simulink model "test_ecef"  (R2019b)
settings: Solver=VariableStepAuto  StartTime=0.0  StopTime=10.0  RelTol=1e-3
settings Model: Creator=markwilkinson  LastModifiedBy=markwilkinson

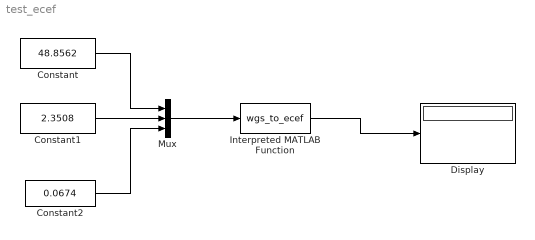
== system test_ecef ==
  Constant : Constant  Value=48.8562
  Constant1 : Constant  Value=2.3508
  Constant2 : Constant  Value=0.0674
  Display : Display
  Interpreted MATLAB Function : MATLABFcn  MATLABFcn=wgs_to_ecef
  Mux : Mux  Inputs=3
  wires:
  Mux/1 -> Interpreted MATLAB Function/1
  Interpreted MATLAB Function/1 -> Display/1
  Constant1/1 -> Mux/2
  Constant2/1 -> Mux/3
  Constant/1 -> Mux/1
